simulink model "car_speed_control_uart"  (R2024b)
settings: Solver=FixedStepAuto  StartTime=0.0  StopTime=50  RelTol=1e-3
libraries: arduinolib x2, simulink_extras x1
settings Model: ExtModeTrigDuration=2  Creator=USER  LastModifiedBy=USER
settings SolverCC: AutoInsertRateTranBlk=on
settings OptimizationCC: EnhancedBackFolding=on  PassReuseOutputArgsAs=Individual arguments  ZeroExternalMemoryAtStartup=off  ZeroInternalMemoryAtStartup=off  MaxStackSize=64  OptimizeBlockOrder=speed  DifferentSizesBufferReuse=on  OptimizationCustomize=off  EfficientTunableParamExpr=on
settings DebuggingCC: ParameterTunabilityLossMsg=error
settings HardwareCC: ProdBitPerInt=16  ProdBitPerPointer=16  ProdBitPerSizeT=16  ProdBitPerPtrDiffT=16  ProdLargestAtomicFloat=None  ProdWordSize=8  ProdHWDeviceType=Atmel->AVR
settings SFSimCC: MATLABDynamicMemAlloc=off
settings RTWCC: Description=Embedded Coder  SystemTargetFile=ert.tlc  HardwareBoard=Arduino Mega 2560  TemplateMakefile=ert_default_tmf  Toolchain=Arduino AVR
settings CodeAppCC: ForceParamTrailComments=on  IgnoreCustomStorageClasses=off  OperatorAnnotations=on  SimulinkDataObjDesc=on  SFDataObjDesc=on  InsertBlockDesc=on
settings ERTTargetCC: SupportContinuousTime=on  SupportVariableSizeSignals=on  ExtModeTransport=3  ExtModeStaticAlloc=on  ExtModeAutomaticAllocSize=off  ExtModeStaticAllocSize=2048  ExtModeMexFile=ext_xcp  ExtModeIntrfLevel=Level2 - Open  InlinedParameterPlacement=Hierarchical

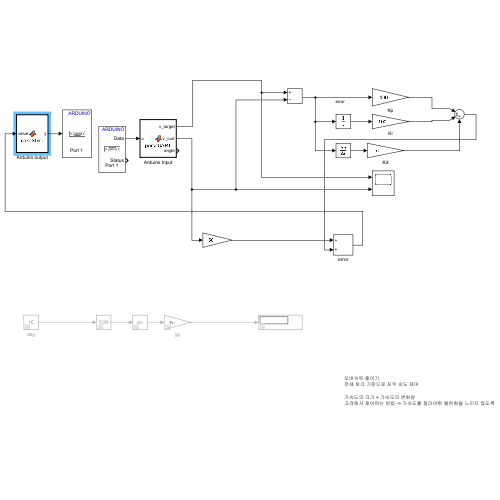
[thumbnail: Simulink's stored preview of the top-level diagram]
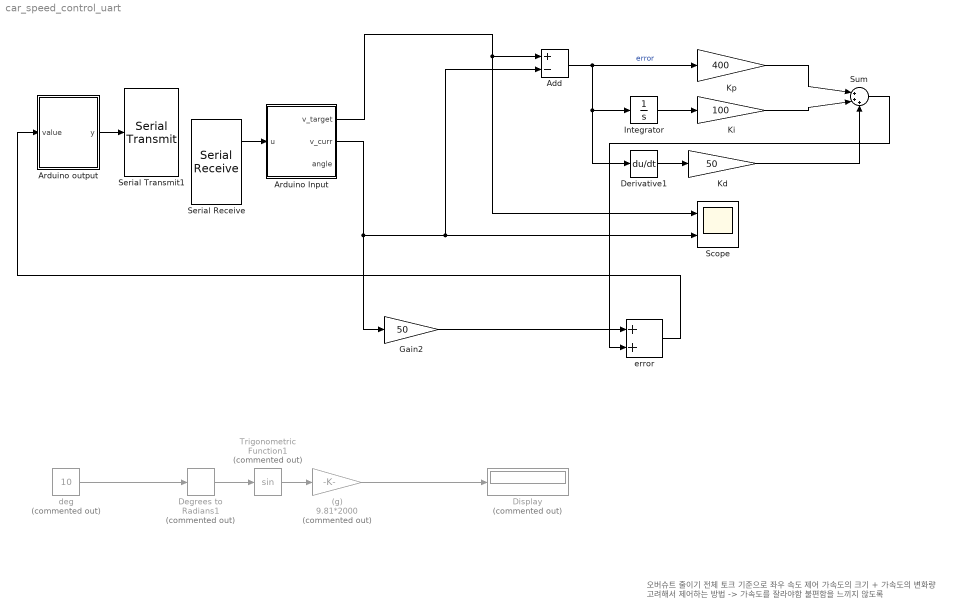
== system car_speed_control_uart ==
  note: 오버슈트 줄이기
      | 전체 토크 기준으로 좌우 속도 제어
      |
      | 가속도의 크기 + 가속도의 변화량
      | 고려해서 제어하는 방법 -> 가속도를 잘라야함 불편함을 느끼지 않도록
  (g) : Gain  Commented=on  Gain=9.81*2000
  Add : Sum  Inputs=+-
  Arduino Input : MATLAB Function  TreatAsAtomicUnit=on
  Arduino output : MATLAB Function  TreatAsAtomicUnit=on
  Degrees to Radians1 : simulink_extras/Transformations/Degrees to Radians  Commented=on
  Derivative1 : Derivative
  Display : Display  Commented=on
  Gain2 : Gain  Gain=50
  Integrator : Integrator
  Kd : Gain  Gain=50
  Ki : Gain  Gain=100
  Kp : Gain  Gain=400
  Scope : Scope  NumInputPorts=2
  Serial Receive : arduinolib/Serial Receive  portNumber=1  DataType=int16  blockPlatform=ARDUINO  TimeOut=0  MaxDataLength=10  isARMArch=off  DataLengthOption=Length via dialog  Datalength=1  Header=[]  Terminator=[]  SampleTime=0.1  ShowOutStatus=on
      settings: SourceProductName=Common
  Serial Transmit1 : arduinolib/Serial Transmit  portNumber=1  sendmode=write  sendformat=Decimal  floatprecision=2  header=[]  terminator=[]  blockPlatform=ARDUINO
      settings: SourceProductName=Common
  Sum : Sum  Inputs=|+++
  Trigonometric Function1 : Trigonometry  Commented=on
  deg : Constant  Commented=on  Value=10
  error : Sum
  wires:
  Arduino Input/2(v_curr) -> Gain2/1, Add/2, Scope/2
  Arduino Input/1(v_target) -> Add/1, Scope/1
  Add/1 -> Derivative1/1, Integrator/1, Kp/1  "error"
  Gain2/1 -> error/1
  error/1 -> Arduino output/1(value)
  deg/1 -> Degrees to Radians1/1
  Degrees to Radians1/1 -> Trigonometric Function1/1
  Trigonometric Function1/1 -> (g)/1
  (g)/1 -> Display/1
  Integrator/1 -> Ki/1
  Derivative1/1 -> Kd/1
  Kp/1 -> Sum/1
  Ki/1 -> Sum/2
  Kd/1 -> Sum/3
  Sum/1 -> error/2
  Serial Receive/1 -> Arduino Input/1(u)
  Arduino output/1(y) -> Serial Transmit1/1

== matlab function car_speed_control_uart/Arduino Input ==
  data: v_target output; u input; v_curr output; angle output
function [v_target, v_curr, angle] = parseUART(u)
    str = char(u);    % uint8 → char
    v_target = 0;
    v_curr = 0;
    angle = 0;

    idxs = find(str == ',');
    if length(idxs) >= 2
        idx1 = idxs(1);
        idx2 = idxs(2);

        s1 = str(1:idx1-1);
        s2 = str(idx1+1:idx2-1);
        s3 = str(idx2+1:end);

        v_target = real(str2double(s1));
        v_curr   = real(str2double(s2));
        angle    = real(str2double(s3)); % 복소수가 아닌 실수임을 명시`
    end
end

== matlab function car_speed_control_uart/Arduino output ==
  data: value input; y output
function y = makeString(value)
    y = zeros(16,1,'uint8');  % 고정 크기 16 byte
    int_part = floor(value);               % 정수부
    frac_part = floor(mod(value*100, 100)); % 소수점 둘째자리까지

    % 수동 ASCII 문자 조합
    y(1) = uint8(floor(int_part/10) + 48);   % 십의 자리
    y(2) = uint8(mod(int_part,10) + 48);     % 일의 자리
    y(3) = uint8('.');                       % 소수점
    y(4) = uint8(floor(frac_part/10) + 48);  % 소수 첫째 자리
    y(5) = uint8(mod(frac_part,10) + 48);    % 소수 둘째 자리
    y(6) = uint8(10);                      % 개행문자
end
